simulink model "energy_storage"  (R2018a)
settings: Solver=ode4  StartTime=0.0  StopTime=simu.tTotal  FixedStep=simu.tStep  RelTol=1e-3
undefined symbols (not defined in the file or in its folder): D11, Delta, DiscIntNeverNeededParam, es1, es2, ess, flex, grid, gsc, gt1, ld, sim, simu, u0, Vbase, vsc, WT
libraries: powerlib x40, pwrsys x37, simulink x2, powerlib_meascontrol x2, simulink_extras x1, sps_avr x1
(part 2 of 2)

== system energy_storage/Wind Farm/Wind Model Kaimal spectrum according to IEC61400-1 ==
  avg_wind : Inport
  Fcn : Fcn  Expr=turb_int*sqrt(L*u(1))/100/sqrt(2)
  Kaimal Filter : Subsystem
  Product : Product  SaturateOnIntegerOverflow=on  OutDataTypeStr=Inherit: Same as first input
  Sum2 : Sum  SaturateOnIntegerOverflow=on  InputSameDT=on  OutDataTypeStr=Inherit: Same as first input
  White Noise_1 : Subsystem  mask(Continuous White Noise.){Cov=[1], Ts=T_sample, seed=256}
      mask prompts: Cov "Noise Power:"; Ts "Sample Time:"
      mask help:
      | White noise for continuous (s-domain) systems.
      | Band-limited using zero-order-hold.
      mask init:
      | r = rand(1,12); r2 = [r(1),r;r,r(12)]; t =[1:13;1:13];
      mask Help: Implemented using white noise into Zero-Order Hold block. The seed and power can be vectors of the same length to produce a vector of white noise sources. For faster simulation, set sample time to the highest value possible but in accordance with the fastest dynamics of system.
      mask Display: plot(t(:),r2(:))
  wind : Outport  InitialOutput=[u0]
  wires:
  Product/1 -> Sum2/1
  Sum2/1 -> wind/1  "wind"
  White Noise_1/1(Out_1) -> Kaimal Filter/2(In)
  Fcn/1 -> Product/1
  Kaimal Filter/1(Out) -> Product/2
  avg_wind/1 -> Sum2/2, Fcn/1, Kaimal Filter/1(avg_wind)

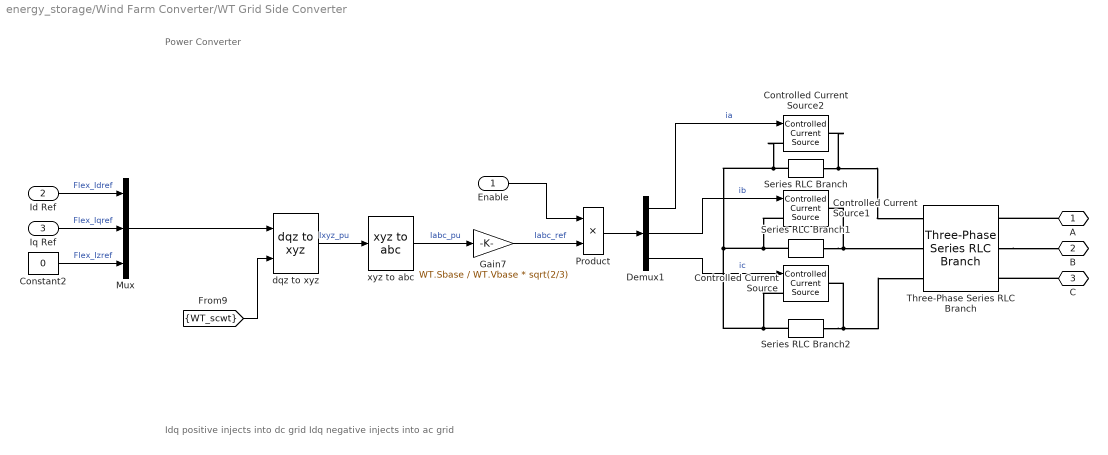
== system energy_storage/Wind Farm Converter/WT Grid Side Converter ==
  note: Power Converter
  note: Idq positive injects into dc grid
      | Idq negative injects into ac grid
  Enable : Inport
  Id Ref : Inport  Port=2
  Iq Ref : Inport  Port=3
  Constant2 : Constant  Value=0
  Controlled Current Source : powerlib/Electrical Sources/Controlled Current Source  Initialize=off  Source_Type=AC  Amplitude=0  Phase=0  Frequency=grid.fn  Measurements=None
  Controlled Current Source1 : powerlib/Electrical Sources/Controlled Current Source  Initialize=off  Source_Type=AC  Amplitude=0  Phase=0  Frequency=grid.fn  Measurements=None
  Controlled Current Source2 : powerlib/Electrical Sources/Controlled Current Source  Initialize=off  Source_Type=AC  Amplitude=0  Phase=0  Frequency=grid.fn  Measurements=None
  Demux1 : Demux  Outputs=3
  Gain7 : Gain  Gain=WT.Sbase / WT.Vbase * sqrt(2/3)
  Mux : Mux  Inputs=3
  Product : Product
  Series RLC Branch : powerlib/Elements/Series RLC Branch  LConnTagsString=__new0  RConnTagsString=__new0  BranchType=RC  Resistance=1e3  Inductance=1e-3  SetiL0=off  InitialCurrent=0  Capacitance=1e3  Setx0=off  InitialVoltage=0  Measurements=None
  Series RLC Branch1 : powerlib/Elements/Series RLC Branch  LConnTagsString=__new0  RConnTagsString=__new0  BranchType=RC  Resistance=1e3  Inductance=1e-3  SetiL0=off  InitialCurrent=0  Capacitance=1e3  Setx0=off  InitialVoltage=0  Measurements=None
  Series RLC Branch2 : powerlib/Elements/Series RLC Branch  LConnTagsString=__new0  RConnTagsString=__new0  BranchType=RC  Resistance=1e3  Inductance=1e-3  SetiL0=off  InitialCurrent=0  Capacitance=1e3  Setx0=off  InitialVoltage=0  Measurements=None
  Three-Phase Series RLC Branch : powerlib/Elements/Three-Phase Series RLC Branch  LConnTagsString=A|B|C  RConnTagsString=A|B|C  BranchType=RL  Resistance=flex.filter.Rac  Inductance=flex.filter.Lac  Capacitance=1e-6  Measurements=None
  dqz to xyz : pwrsys/Transformations/dqz to xyz  SystemSampleTime=-1
      settings: SourceProductName=NTNU Power Systems
  xyz to abc : pwrsys/Transformations/xyz to abc  typeTransf=Amplitude-invariant
      settings: SourceProductName=NTNU Power Systems
  A : PMIOPort  Side=Right
  B : PMIOPort  Port=2  Side=Right
  C : PMIOPort  Port=3  Side=Right
  wires:
  [WT_scwt] -> dqz to xyz/2
  xyz to abc/1 -> Gain7/1  "Iabc_pu"
  Gain7/1 -> Product/2  "Iabc_ref"
  dqz to xyz/1 -> xyz to abc/1  "Ixyz_pu"
  Enable/1 -> Product/1
  Id Ref/1 -> Mux/1  "Flex_Idref"
  Iq Ref/1 -> Mux/2  "Flex_Iqref"
  Constant2/1 -> Mux/3  "Flex_Izref"
  Mux/1 -> dqz to xyz/1
  Demux1/1 -> Controlled Current Source2/1  "ia"
  Demux1/2 -> Controlled Current Source1/1  "ib"
  Product/1 -> Demux1/1
  Demux1/3 -> Controlled Current Source/1  "ic"
  connections:
  Controlled Current Source/RConn1 -- Series RLC Branch2/LConn1 -- Three-Phase Series RLC Branch/RConn3
  Controlled Current Source2/RConn1 -- Series RLC Branch/LConn1 -- Three-Phase Series RLC Branch/RConn1
  Controlled Current Source1/RConn1 -- Series RLC Branch1/LConn1 -- Three-Phase Series RLC Branch/RConn2
  Controlled Current Source/LConn1 -- Series RLC Branch2/RConn1 -- Series RLC Branch1/RConn1 -- Controlled Current Source1/LConn1 -- Controlled Current Source2/LConn1 -- Series RLC Branch/RConn1
  A/RConn1 -- Three-Phase Series RLC Branch/LConn1
  C/RConn1 -- Three-Phase Series RLC Branch/LConn3
  Three-Phase Series RLC Branch/LConn2 -- B/RConn1

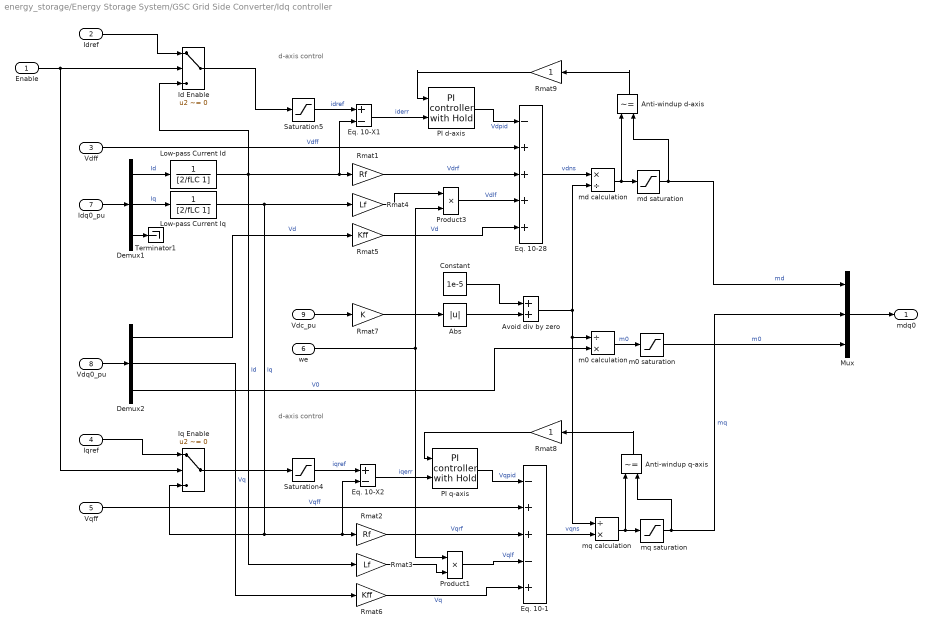
== system energy_storage/Energy Storage System/GSC Grid Side Converter/Idq controller ==
  note: d-axis control
  note: d-axis control
  Enable : Inport
  Idref : Inport  Port=2
  Vdff : Inport  Port=3
  Iqref : Inport  Port=4
  Vqff : Inport  Port=5
  we : Inport  Port=6
  Idq0_pu : Inport  Port=7
  Vdq0_pu : Inport  Port=8
  Vdc_pu : Inport  Port=9
  Abs : Abs  ZeroCross=off
  Anti-windup d-axis : RelationalOperator  Operator=~=  OutDataTypeStr=boolean  RndMeth=Simplest
  Anti-windup q-axis : RelationalOperator  Operator=~=  OutDataTypeStr=boolean  RndMeth=Simplest
  Avoid div by zero : Sum
  Constant : Constant  Value=1e-5
  Demux1 : Demux  Outputs=3
  Demux2 : Demux  Outputs=3
  Eq. 10-1 : Sum  Inputs=-++-+  SaturateOnIntegerOverflow=on  InputSameDT=on  OutDataTypeStr=Inherit: Same as first input
  Eq. 10-28 : Sum  Inputs=-++++  SaturateOnIntegerOverflow=on  InputSameDT=on  OutDataTypeStr=Inherit: Same as first input
  Eq. 10-X1 : Sum  Inputs=+-  SaturateOnIntegerOverflow=on  InputSameDT=on  OutDataTypeStr=Inherit: Same as first input
  Eq. 10-X2 : Sum  Inputs=+-  SaturateOnIntegerOverflow=on  InputSameDT=on  OutDataTypeStr=Inherit: Same as first input
  Id Enable : Switch  Criteria=u2 ~= 0
  Iq Enable : Switch  Criteria=u2 ~= 0
  Low-pass Current Id : TransferFcn  Denominator=[2/fLC 1]
  Low-pass Current Iq : TransferFcn  Denominator=[2/fLC 1]
  Mux : Mux  Inputs=3
  PI d-axis : pwrsys/Controllers/PI controller  with Hold  Kp=kp  Ki=ki  Max=K*mmax  Min=-K*mmax  x0=0  Ts=Ts
      settings: SourceProductName=NTNU Power Systems
  PI q-axis : pwrsys/Controllers/PI controller  with Hold  Kp=kp  Ki=ki  Max=K*mmax  Min=-K*mmax  x0=0  Ts=Ts
      settings: SourceProductName=NTNU Power Systems
  Product1 : Product  SaturateOnIntegerOverflow=on  RndMeth=Zero  InputSameDT=on  OutDataTypeStr=Inherit: Same as first input
  Product3 : Product  SaturateOnIntegerOverflow=on  RndMeth=Zero  InputSameDT=on  OutDataTypeStr=Inherit: Same as first input
  Rmat1 : Gain  Gain=Rf
  Rmat2 : Gain  Gain=Rf
  Rmat3 : Gain  Gain=Lf
  Rmat4 : Gain  Gain=Lf
  Rmat5 : Gain  Gain=Kff
  Rmat6 : Gain  Gain=Kff
  Rmat7 : Gain  Gain=K
  Rmat8 : Gain
  Rmat9 : Gain
  Saturation4 : Saturate  UpperLimit=Imax  LowerLimit=-Imax
  Saturation5 : Saturate  UpperLimit=Imax  LowerLimit=-Imax
  Terminator1 : Terminator
  m0 saturation : Saturate  UpperLimit=mmax  LowerLimit=-mmax
  m0 calculation : Product  Inputs=/*
  md calculation : Product  Inputs=*/
  md saturation : Saturate  UpperLimit=mmax  LowerLimit=-mmax
  mq saturation : Saturate  UpperLimit=mmax  LowerLimit=-mmax
  mq calculation : Product  Inputs=/*
  mdq0 : Outport
  wires:
  Idref/1 -> Id Enable/1
  Iqref/1 -> Iq Enable/1
  Demux1/3 -> Terminator1/1
  Vdq0_pu/1 -> Demux2/1
  Mux/1 -> mdq0/1
  Demux2/3 -> m0 calculation/2  "V0"
  Product3/1 -> Eq. 10-28/4  "Vdlf"
  Rmat4/1 -> Product3/1
  md saturation/1 -> Anti-windup d-axis/2, Mux/1  "md"
  Anti-windup d-axis/1 -> Rmat9/1
  PI d-axis/1 -> Eq. 10-28/1  "Vdpid"
  Eq. 10-28/1 -> md calculation/1  "vdns"
  Saturation5/1 -> Eq. 10-X1/1  "idref"
  Demux2/1 -> Rmat5/1  "Vd"
  Rmat5/1 -> Eq. 10-28/5  "Vd"
  Vdff/1 -> Eq. 10-28/2  "Vdff"
  Demux1/2 -> Low-pass Current Iq/1  "Iq"
  Rmat6/1 -> Eq. 10-1/5  "Vq"
  Saturation4/1 -> Eq. 10-X2/1  "iqref"
  mq saturation/1 -> Mux/2, Anti-windup q-axis/2  "mq"
  Rmat3/1 -> Product1/2
  Anti-windup q-axis/1 -> Rmat8/1
  Demux1/1 -> Low-pass Current Id/1  "Id"
  Vqff/1 -> Eq. 10-1/2  "Vqff"
  Eq. 10-1/1 -> mq calculation/2  "vqns"
  Demux2/2 -> Rmat6/1  "Vq"
  Product1/1 -> Eq. 10-1/4  "Vqlf"
  Eq. 10-X2/1 -> PI q-axis/2  "iqerr"
  we/1 -> Product3/2, Product1/1
  PI q-axis/1 -> Eq. 10-1/1  "Vqpid"
  Idq0_pu/1 -> Demux1/1
  Low-pass Current Id/1 -> Id Enable/3, Eq. 10-X1/2, Rmat1/1, Rmat3/1  "Id"
  Low-pass Current Iq/1 -> Iq Enable/3, Eq. 10-X2/2, Rmat2/1, Rmat4/1  "Iq"
  Rmat2/1 -> Eq. 10-1/3  "Vqrf"
  Rmat1/1 -> Eq. 10-28/3  "Vdrf"
  Eq. 10-X1/1 -> PI d-axis/2  "iderr"
  Avoid div by zero/1 -> m0 calculation/1, mq calculation/1, md calculation/2
  Constant/1 -> Avoid div by zero/1
  Abs/1 -> Avoid div by zero/2
  md calculation/1 -> Anti-windup d-axis/1, md saturation/1
  mq calculation/1 -> mq saturation/1, Anti-windup q-axis/1
  m0 calculation/1 -> m0 saturation/1  "m0"
  Vdc_pu/1 -> Rmat7/1
  Rmat7/1 -> Abs/1
  m0 saturation/1 -> Mux/3  "m0"
  Rmat8/1 -> PI q-axis/1
  Rmat9/1 -> PI d-axis/1
  Enable/1 -> Id Enable/2, Iq Enable/2
  Id Enable/1 -> Saturation5/1
  Iq Enable/1 -> Saturation4/1

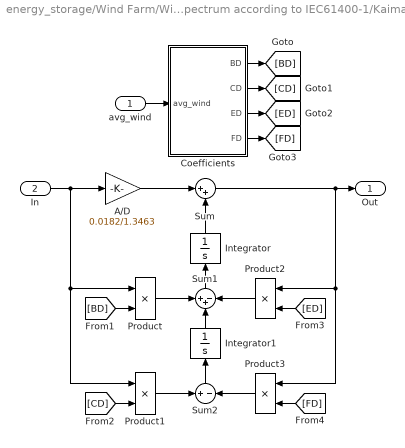
== system energy_storage/Wind Farm/Wind Model Kaimal spectrum according to IEC61400-1/Kaimal Filter ==
  avg_wind : Inport
  In : Inport  Port=2
  A/D : Gain  Gain=0.0182/1.3463  SaturateOnIntegerOverflow=on  OutDataTypeStr=Inherit: Same as input  ParamDataTypeStr=Inherit: Same as input
  Coefficients : Subsystem
  Integrator : Integrator
  Integrator1 : Integrator
  Product{,1..3} (4 alike) : Product  SaturateOnIntegerOverflow=on  OutDataTypeStr=Inherit: Same as first input
  Sum : Sum  Inputs=|++  SaturateOnIntegerOverflow=on
  Sum1 : Sum  Inputs=++-  SaturateOnIntegerOverflow=on
  Sum2 : Sum  Inputs=+|-  SaturateOnIntegerOverflow=on
  Out : Outport
  wires:
  avg_wind/1 -> Coefficients/1(avg_wind)
  Coefficients/4(FD) -> [FD]
  Coefficients/3(ED) -> [ED]
  Coefficients/2(CD) -> [CD]
  Coefficients/1(BD) -> [BD]
  [FD] -> Product3/2
  [ED] -> Product2/2
  [CD] -> Product1/2
  [BD] -> Product/2
  In/1 -> Product1/1, Product/1, A/D/1
  Sum/1 -> Out/1, Product3/1, Product2/1
  Product1/1 -> Sum2/1
  Product3/1 -> Sum2/2
  Sum2/1 -> Integrator1/1
  Product2/1 -> Sum1/3
  Integrator1/1 -> Sum1/2
  Product/1 -> Sum1/1
  Sum1/1 -> Integrator/1
  Integrator/1 -> Sum/2
  A/D/1 -> Sum/1

== system energy_storage/Wind Farm/Wind Model Kaimal spectrum according to IEC61400-1/White Noise_1 ==
  Gain : Gain  Gain=[sqrt(Cov)]/[sqrt(Ts)]  SaturateOnIntegerOverflow=on  OutDataTypeStr=Inherit: Same as input  ParamDataTypeStr=Inherit: Same as input
  White Noise : RandomNumber  Seed=seed  SampleTime=Ts
  Zero-Order Hold : ZeroOrderHold  SampleTime=Ts
  Out_1 : Outport
  wires:
  White Noise/1 -> Zero-Order Hold/1
  Gain/1 -> Out_1/1
  Zero-Order Hold/1 -> Gain/1

== system energy_storage/Wind Farm/Wind Model Kaimal spectrum according to IEC61400-1/Kaimal Filter/Coefficients ==
  avg_wind : Inport
  BD coeff : Fcn  Expr=1.3653/1.3463/(L/2/pi/u(1))
  CD coeff : Fcn  Expr=0.9846/1.3463/(L/2/pi/u(1))^2
  ED coeff : Fcn  Expr=3.7593/1.3463/(L/2/pi/u(1))
  FD coeff : Fcn  Expr=1/1.3463/(L/2/pi/u(1))^2
  BD : Outport
  CD : Outport  Port=2
  ED : Outport  Port=3
  FD : Outport  Port=4
  wires:
  FD coeff/1 -> FD/1
  ED coeff/1 -> ED/1
  CD coeff/1 -> CD/1
  BD coeff/1 -> BD/1
  avg_wind/1 -> FD coeff/1, ED coeff/1, CD coeff/1, BD coeff/1
